simulink model "FrictionIdentification"  (R2013a)
settings: Solver=FixedStepDiscrete  StartTime=0.0  StopTime=60  FixedStep=robot.Ts  RelTol=1e-3
libraries: WBCLibrary x20
settings Model: Creator=Raffaello  LastModifiedBy=Raffaello
settings DataIOCC: LimitDataPoints=off  OutputSaveName=out
settings DebuggingCC: InheritedTsInSrcMsg=none

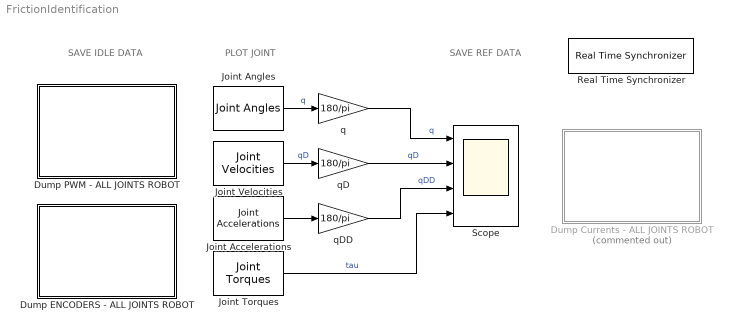
== system FrictionIdentification ==
  note: SAVE
      | IDLE DATA
  note: SAVE
      | REF DATA
  note: PLOT
      | JOINT
  Dump Currents - ALL JOINTS ROBOT : Subsystem  Commented=on  mask{output='getCurrent'}
      mask prompts: output "Output port"
      mask Display:
      | color('red'); plot([10 20 30 40], [10 20 10 15]);
      | color('blue'); plot([10 20 30 40], [15 10 20 12]);
      | color('green'); plot([10 20 30 40], [13 16 12 18]);
  Dump ENCODERS - ALL JOINTS ROBOT : Subsystem  mask{output='getMotorEncoderSpeeds'}
      mask prompts: output "Output port"
      mask Display:
      | color('red'); plot([10 20 30 40], [10 20 10 15]);
      | color('blue'); plot([10 20 30 40], [15 10 20 12]);
      | color('green'); plot([10 20 30 40], [13 16 12 18]);
  Dump PWM - ALL JOINTS ROBOT : Subsystem  mask{output='getOutputs'}
      mask prompts: output "Output port"
      mask Display:
      | color('red'); plot([10 20 30 40], [10 20 10 15]);
      | color('blue'); plot([10 20 30 40], [15 10 20 12]);
      | color('green'); plot([10 20 30 40], [13 16 12 18]);
  Joint Accelerations : WBCLibrary/wholeBodyStates/Joint Accelerations  robotName=robot.robotName  localName=robot.localName
  Joint Angles : WBCLibrary/wholeBodyStates/Joint Angles  robotName=robot.robotName  localName=robot.localName
  Joint Torques : WBCLibrary/wholeBodyStates/Joint Torques  robotName=robot.robotName  localName=robot.localName
  Joint Velocities : WBCLibrary/wholeBodyStates/Joint Velocities  robotName=robot.robotName  localName=robot.localName
  Real Time Synchronizer : WBCLibrary/Utilities/Real Time Synchronizer  Priority=-10  threadPeriod=robot.Ts
  Scope : Scope  NumInputPorts=4
      settings: ShowLegends=on  TimeRange=60  YMin=-15~-5~-20~-7  YMax=15~5~25~6  SaveName=ScopeData2
  q : Gain  Gain=180/pi
  qD : Gain  Gain=180/pi
  qDD : Gain  Gain=180/pi
  wires:
  Joint Angles/1 -> q/1  "q"
  Joint Velocities/1 -> qD/1  "qD"
  Joint Torques/1 -> Scope/4  "tau"
  q/1 -> Scope/1  "q"
  qD/1 -> Scope/2  "qD"
  Joint Accelerations/1 -> qDD/1
  qDD/1 -> Scope/3  "qDD"

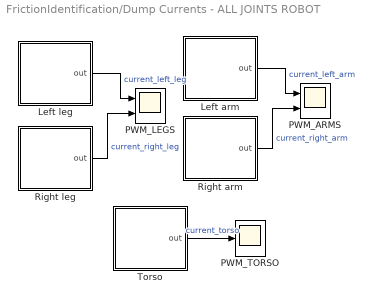
== system FrictionIdentification/Dump Currents - ALL JOINTS ROBOT ==
  Left arm : Subsystem  mask{type_arm='left_arm', output=output}
      mask prompts: type_arm "Type leg"; output "Output Port"
  Left leg : Subsystem  mask{type_arm='left_leg', output=output}
      mask prompts: type_arm "Type leg"; output "Output port"
  PWM_ARMS : Scope  NumInputPorts=2
      settings: TimeRange=60  YMin=-10~-10  YMax=12.5~15
  PWM_LEGS : Scope  NumInputPorts=2
      settings: TimeRange=60  YMin=-10~-10  YMax=12.5~15
  PWM_TORSO : Scope
      settings: TimeRange=60  YMin=-10  YMax=12.5  SaveName=ScopeData5
  Right arm : Subsystem  mask{type_arm='right_arm', output=output}
      mask prompts: type_arm "Type leg"; output "Output Port"
  Right leg : Subsystem  mask{type_arm='right_leg', output=output}
      mask prompts: type_arm "Type leg"; output "Output port"
  Torso : Subsystem  mask{type_arm='torso', output=output}
      mask prompts: type_arm "Type leg"; output "Output port"
  wires:
  Left arm/1(out) -> PWM_ARMS/1  "current_left_arm"
  Right arm/1(out) -> PWM_ARMS/2  "current_right_arm"
  Torso/1(out) -> PWM_TORSO/1  "current_torso"
  Right leg/1(out) -> PWM_LEGS/2  "current_right_leg"
  Left leg/1(out) -> PWM_LEGS/1  "current_left_leg"

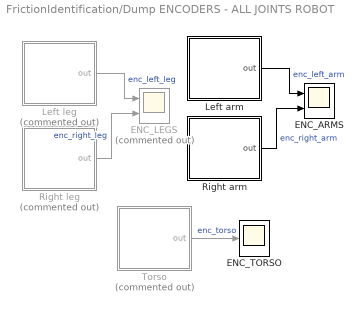
== system FrictionIdentification/Dump ENCODERS - ALL JOINTS ROBOT ==
  ENC_ARMS : Scope  NumInputPorts=2
      settings: TimeRange=60  YMin=-1~-500  YMax=1~450
  ENC_LEGS : Scope  Commented=on  NumInputPorts=2
      settings: TimeRange=60  YMin=-10~-10  YMax=12.5~15
  ENC_TORSO : Scope
      settings: TimeRange=60  YMin=-10  YMax=12.5  SaveName=ScopeData5
  Left arm : Subsystem  mask{type_arm='left_arm', output=output}
      mask prompts: type_arm "Type leg"; output "Output Port"
  Left leg : Subsystem  Commented=on  mask{type_arm='left_leg', output=output}
      mask prompts: type_arm "Type leg"; output "Output port"
  Right arm : Subsystem  mask{type_arm='right_arm', output=output}
      mask prompts: type_arm "Type leg"; output "Output Port"
  Right leg : Subsystem  Commented=on  mask{type_arm='right_leg', output=output}
      mask prompts: type_arm "Type leg"; output "Output port"
  Torso : Subsystem  Commented=on  mask{type_arm='torso', output=output}
      mask prompts: type_arm "Type leg"; output "Output port"
  wires:
  Left arm/1(out) -> ENC_ARMS/1  "enc_left_arm"
  Right arm/1(out) -> ENC_ARMS/2  "enc_right_arm"
  Torso/1(out) -> ENC_TORSO/1  "enc_torso"
  Right leg/1(out) -> ENC_LEGS/2  "enc_right_leg"
  Left leg/1(out) -> ENC_LEGS/1  "enc_left_leg"

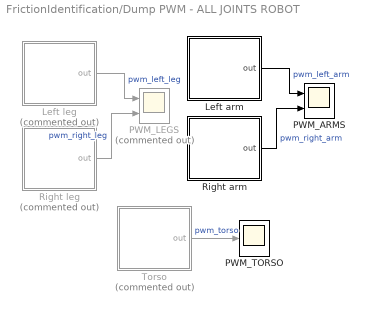
== system FrictionIdentification/Dump PWM - ALL JOINTS ROBOT ==
  Left arm : Subsystem  mask{type_arm='left_arm', output=output}
      mask prompts: type_arm "Type leg"; output "Output Port"
  Left leg : Subsystem  Commented=on  mask{type_arm='left_leg', output=output}
      mask prompts: type_arm "Type leg"; output "Output port"
  PWM_ARMS : Scope  NumInputPorts=2
      settings: TimeRange=60  YMin=-500~-10  YMax=1000~15
  PWM_LEGS : Scope  Commented=on  NumInputPorts=2
      settings: TimeRange=60  YMin=-10~-10  YMax=12.5~15
  PWM_TORSO : Scope
      settings: TimeRange=60  YMin=-10  YMax=12.5  SaveName=ScopeData5
  Right arm : Subsystem  mask{type_arm='right_arm', output=output}
      mask prompts: type_arm "Type leg"; output "Output Port"
  Right leg : Subsystem  Commented=on  mask{type_arm='right_leg', output=output}
      mask prompts: type_arm "Type leg"; output "Output port"
  Torso : Subsystem  Commented=on  mask{type_arm='torso', output=output}
      mask prompts: type_arm "Type leg"; output "Output port"
  wires:
  Left arm/1(out) -> PWM_ARMS/1  "pwm_left_arm"
  Right arm/1(out) -> PWM_ARMS/2  "pwm_right_arm"
  Torso/1(out) -> PWM_TORSO/1  "pwm_torso"
  Right leg/1(out) -> PWM_LEGS/2  "pwm_right_leg"
  Left leg/1(out) -> PWM_LEGS/1  "pwm_left_leg"

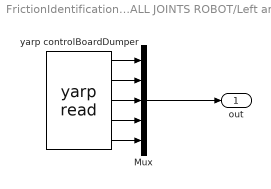
== system FrictionIdentification/Dump Currents - ALL JOINTS ROBOT/Left arm ==
  Mux : Mux  Inputs=5
  yarp controlBoardDumper : WBCLibrary/Utilities/yarp read  from=['/controlBoardDumper/' type_arm '/' output]  to='...'  num=5  blocking=off  timestamp=off  autoconnect=on
  out : Outport
  wires:
  Mux/1 -> out/1
  yarp controlBoardDumper/1 -> Mux/1
  yarp controlBoardDumper/3 -> Mux/3
  yarp controlBoardDumper/2 -> Mux/2
  yarp controlBoardDumper/5 -> Mux/5
  yarp controlBoardDumper/4 -> Mux/4

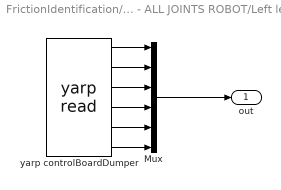
== system FrictionIdentification/Dump Currents - ALL JOINTS ROBOT/Left leg ==
  Mux : Mux  Inputs=6
  yarp controlBoardDumper : WBCLibrary/Utilities/yarp read  from=['/controlBoardDumper/' type_arm '/' output]  to='...'  num=6  blocking=off  timestamp=off  autoconnect=on
  out : Outport
  wires:
  Mux/1 -> out/1
  yarp controlBoardDumper/1 -> Mux/1
  yarp controlBoardDumper/3 -> Mux/3
  yarp controlBoardDumper/2 -> Mux/2
  yarp controlBoardDumper/5 -> Mux/5
  yarp controlBoardDumper/6 -> Mux/6
  yarp controlBoardDumper/4 -> Mux/4

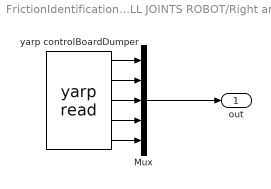
== system FrictionIdentification/Dump Currents - ALL JOINTS ROBOT/Right arm ==
  Mux : Mux  Inputs=5
  yarp controlBoardDumper : WBCLibrary/Utilities/yarp read  from=['/controlBoardDumper/' type_arm '/' output]  to='...'  num=5  blocking=off  timestamp=off  autoconnect=on
  out : Outport
  wires:
  Mux/1 -> out/1
  yarp controlBoardDumper/1 -> Mux/1
  yarp controlBoardDumper/3 -> Mux/3
  yarp controlBoardDumper/2 -> Mux/2
  yarp controlBoardDumper/5 -> Mux/5
  yarp controlBoardDumper/4 -> Mux/4

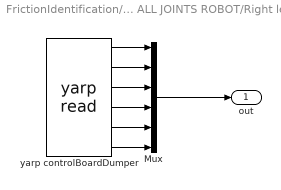
== system FrictionIdentification/Dump Currents - ALL JOINTS ROBOT/Right leg ==
  Mux : Mux  Inputs=6
  yarp controlBoardDumper : WBCLibrary/Utilities/yarp read  from=['/controlBoardDumper/' type_arm '/' output]  to='...'  num=6  blocking=off  timestamp=off  autoconnect=on
  out : Outport
  wires:
  Mux/1 -> out/1
  yarp controlBoardDumper/1 -> Mux/1
  yarp controlBoardDumper/3 -> Mux/3
  yarp controlBoardDumper/2 -> Mux/2
  yarp controlBoardDumper/5 -> Mux/5
  yarp controlBoardDumper/6 -> Mux/6
  yarp controlBoardDumper/4 -> Mux/4

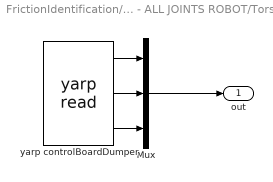
== system FrictionIdentification/Dump Currents - ALL JOINTS ROBOT/Torso ==
  Mux : Mux  Inputs=3
  yarp controlBoardDumper : WBCLibrary/Utilities/yarp read  from=['/controlBoardDumper/' type_arm '/' output]  to='...'  num=3  blocking=off  timestamp=off  autoconnect=on
  out : Outport
  wires:
  Mux/1 -> out/1
  yarp controlBoardDumper/1 -> Mux/1
  yarp controlBoardDumper/3 -> Mux/3
  yarp controlBoardDumper/2 -> Mux/2

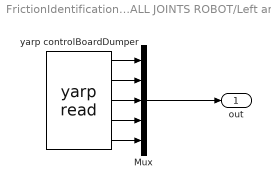
== system FrictionIdentification/Dump ENCODERS - ALL JOINTS ROBOT/Left arm ==
  Mux : Mux  Inputs=5
  yarp controlBoardDumper : WBCLibrary/Utilities/yarp read  from=['/controlBoardDumper/' type_arm '/' output]  to='...'  num=5  blocking=off  timestamp=off  autoconnect=on
  out : Outport
  wires:
  Mux/1 -> out/1
  yarp controlBoardDumper/1 -> Mux/1
  yarp controlBoardDumper/3 -> Mux/3
  yarp controlBoardDumper/2 -> Mux/2
  yarp controlBoardDumper/5 -> Mux/5
  yarp controlBoardDumper/4 -> Mux/4

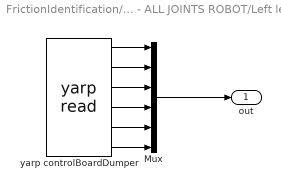
== system FrictionIdentification/Dump ENCODERS - ALL JOINTS ROBOT/Left leg ==
  Mux : Mux  Inputs=6
  yarp controlBoardDumper : WBCLibrary/Utilities/yarp read  from=['/controlBoardDumper/' type_arm '/' output]  to='...'  num=6  blocking=off  timestamp=off  autoconnect=on
  out : Outport
  wires:
  Mux/1 -> out/1
  yarp controlBoardDumper/1 -> Mux/1
  yarp controlBoardDumper/3 -> Mux/3
  yarp controlBoardDumper/2 -> Mux/2
  yarp controlBoardDumper/5 -> Mux/5
  yarp controlBoardDumper/6 -> Mux/6
  yarp controlBoardDumper/4 -> Mux/4

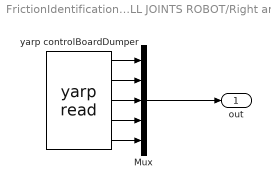
== system FrictionIdentification/Dump ENCODERS - ALL JOINTS ROBOT/Right arm ==
  Mux : Mux  Inputs=5
  yarp controlBoardDumper : WBCLibrary/Utilities/yarp read  from=['/controlBoardDumper/' type_arm '/' output]  to='...'  num=5  blocking=off  timestamp=off  autoconnect=on
  out : Outport
  wires:
  Mux/1 -> out/1
  yarp controlBoardDumper/1 -> Mux/1
  yarp controlBoardDumper/3 -> Mux/3
  yarp controlBoardDumper/2 -> Mux/2
  yarp controlBoardDumper/5 -> Mux/5
  yarp controlBoardDumper/4 -> Mux/4

== system FrictionIdentification/Dump ENCODERS - ALL JOINTS ROBOT/Right leg ==
  Mux : Mux  Inputs=6
  yarp controlBoardDumper : WBCLibrary/Utilities/yarp read  from=['/controlBoardDumper/' type_arm '/' output]  to='...'  num=6  blocking=off  timestamp=off  autoconnect=on
  out : Outport
  wires:
  Mux/1 -> out/1
  yarp controlBoardDumper/1 -> Mux/1
  yarp controlBoardDumper/3 -> Mux/3
  yarp controlBoardDumper/2 -> Mux/2
  yarp controlBoardDumper/5 -> Mux/5
  yarp controlBoardDumper/6 -> Mux/6
  yarp controlBoardDumper/4 -> Mux/4

== system FrictionIdentification/Dump ENCODERS - ALL JOINTS ROBOT/Torso ==
  Mux : Mux  Inputs=3
  yarp controlBoardDumper : WBCLibrary/Utilities/yarp read  from=['/controlBoardDumper/' type_arm '/' output]  to='...'  num=3  blocking=off  timestamp=off  autoconnect=on
  out : Outport
  wires:
  Mux/1 -> out/1
  yarp controlBoardDumper/1 -> Mux/1
  yarp controlBoardDumper/3 -> Mux/3
  yarp controlBoardDumper/2 -> Mux/2

== system FrictionIdentification/Dump PWM - ALL JOINTS ROBOT/Left arm ==
  Mux : Mux  Inputs=5
  yarp controlBoardDumper : WBCLibrary/Utilities/yarp read  from=['/controlBoardDumper/' type_arm '/' output]  to='...'  num=5  blocking=off  timestamp=off  autoconnect=on
  out : Outport
  wires:
  Mux/1 -> out/1
  yarp controlBoardDumper/1 -> Mux/1
  yarp controlBoardDumper/3 -> Mux/3
  yarp controlBoardDumper/2 -> Mux/2
  yarp controlBoardDumper/5 -> Mux/5
  yarp controlBoardDumper/4 -> Mux/4

== system FrictionIdentification/Dump PWM - ALL JOINTS ROBOT/Left leg ==
  Mux : Mux  Inputs=6
  yarp controlBoardDumper : WBCLibrary/Utilities/yarp read  from=['/controlBoardDumper/' type_arm '/' output]  to='...'  num=6  blocking=off  timestamp=off  autoconnect=on
  out : Outport
  wires:
  Mux/1 -> out/1
  yarp controlBoardDumper/1 -> Mux/1
  yarp controlBoardDumper/3 -> Mux/3
  yarp controlBoardDumper/2 -> Mux/2
  yarp controlBoardDumper/5 -> Mux/5
  yarp controlBoardDumper/6 -> Mux/6
  yarp controlBoardDumper/4 -> Mux/4

== system FrictionIdentification/Dump PWM - ALL JOINTS ROBOT/Right arm ==
  Mux : Mux  Inputs=5
  yarp controlBoardDumper : WBCLibrary/Utilities/yarp read  from=['/controlBoardDumper/' type_arm '/' output]  to='...'  num=5  blocking=off  timestamp=off  autoconnect=on
  out : Outport
  wires:
  Mux/1 -> out/1
  yarp controlBoardDumper/1 -> Mux/1
  yarp controlBoardDumper/3 -> Mux/3
  yarp controlBoardDumper/2 -> Mux/2
  yarp controlBoardDumper/5 -> Mux/5
  yarp controlBoardDumper/4 -> Mux/4

== system FrictionIdentification/Dump PWM - ALL JOINTS ROBOT/Right leg ==
  Mux : Mux  Inputs=6
  yarp controlBoardDumper : WBCLibrary/Utilities/yarp read  from=['/controlBoardDumper/' type_arm '/' output]  to='...'  num=6  blocking=off  timestamp=off  autoconnect=on
  out : Outport
  wires:
  Mux/1 -> out/1
  yarp controlBoardDumper/1 -> Mux/1
  yarp controlBoardDumper/3 -> Mux/3
  yarp controlBoardDumper/2 -> Mux/2
  yarp controlBoardDumper/5 -> Mux/5
  yarp controlBoardDumper/6 -> Mux/6
  yarp controlBoardDumper/4 -> Mux/4

== system FrictionIdentification/Dump PWM - ALL JOINTS ROBOT/Torso ==
  Mux : Mux  Inputs=3
  yarp controlBoardDumper : WBCLibrary/Utilities/yarp read  from=['/controlBoardDumper/' type_arm '/' output]  to='...'  num=3  blocking=off  timestamp=off  autoconnect=on
  out : Outport
  wires:
  Mux/1 -> out/1
  yarp controlBoardDumper/1 -> Mux/1
  yarp controlBoardDumper/3 -> Mux/3
  yarp controlBoardDumper/2 -> Mux/2
